simulink model "all_sys_sim"  (R2014a)
settings: Solver=ode45  StartTime=0.0  StopTime=10.0  RelTol=1e-3
values from neighbouring files (symbols this model uses):
  beam_sys = sys_class    [create_all_sys.m]
  build_sys = sys_class    [create_all_sys.m]
  fom_sys = sys_class    [create_all_sys.m]
  heat_sys = sys_class    [create_all_sys.m]
  heli_sys = sys_class    [create_all_sys.m]
  iss_sys = sys_class    [create_all_sys.m]
  mcs_sys = sys_class    [create_all_sys.m]
  MNA1_sys = sys_class    [create_all_sys.m]
  MNA5_sys = sys_class    [create_all_sys.m]
  pde_sys = sys_class    [create_all_sys.m]
  tline_sys = sys_class    [create_all_sys.m]
settings Model: Creator=UX31  LastModifiedBy=UX31

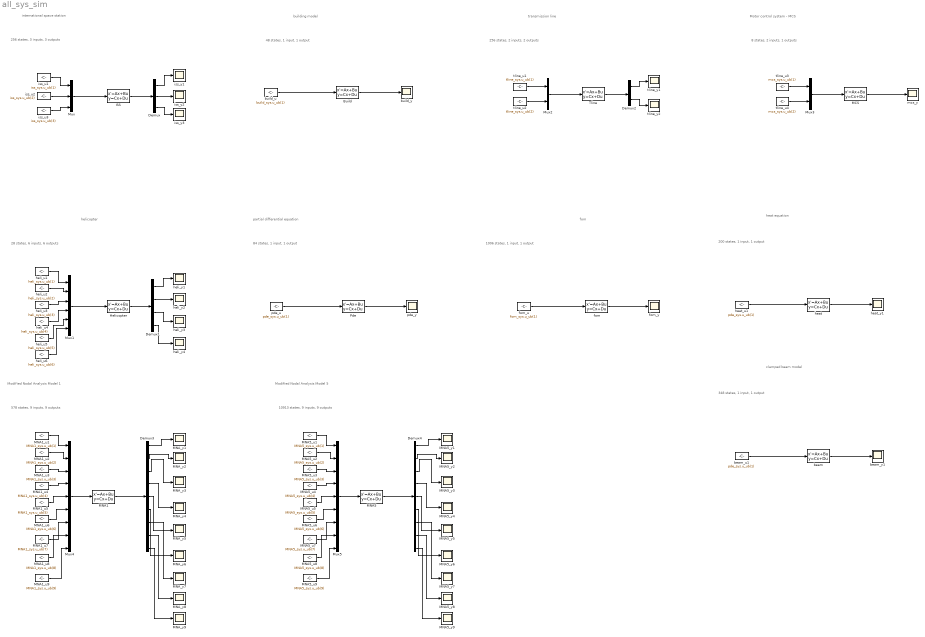
== system all_sys_sim ==
  note: 48 states, 1 input, 1 output
  note: 256 states, 3 inputs, 3 outputs
  note: 84 states, 1 input, 1 output
  note: 28 states, 6 inputs, 6 outputs
  note: 256 states, 2 inputs, 2 outputs
  note: 1006 states, 1 input, 1 output
  note: international space station
  note: building model
  note: helicopter
  note: partial differential equation
  note: fom
  note: transmission line
  note: 8 states, 2 inputs, 1 outputs
  note: Motor control system - MCS
  note: 578 states, 9 inputs, 9 outputs
  note: Modified Nodal Analysis Model 1
  note: 10913 states, 9 inputs, 9 outputs
  note: Modified Nodal Analysis Model 5
  note: 200 states, 1 input, 1 output
  note: heat equation
  note: 348 states, 1 input, 1 output
  note: clamped beam model
  Build : StateSpace  A=build_sys.sys.a  B=build_sys.sys.b  C=build_sys.sys.c  D=build_sys.sys.d  X0=build_sys.x0_lb
  Demux : Demux  Outputs=3
  Demux1 : Demux
  Demux2 : Demux  Outputs=2
  Demux3 : Demux  Outputs=9
  Demux4 : Demux  Outputs=9
  Helicopter : StateSpace  A=heli_sys.sys.a  B=heli_sys.sys.b  C=heli_sys.sys.c  D=heli_sys.sys.d  X0=heli_sys.x0_lb
  ISS : StateSpace  A=iss_sys.sys.a  B=iss_sys.sys.b  C=iss_sys.sys.c  D=iss_sys.sys.d  X0=iss_sys.x0_lb
  MCS : StateSpace  A=mcs_sys.sys.a  B=mcs_sys.sys.b  C=mcs_sys.sys.c  D=mcs_sys.sys.d  X0=mcs_sys.x0_lb
  MNA1 : StateSpace  A=MNA1_sys.sys.a  B=MNA1_sys.sys.b  C=MNA1_sys.sys.c  D=MNA1_sys.sys.d  X0=MNA1_sys.x0_lb
  MNA1_u1 : Constant  Value=MNA1_sys.u_ub(1)
  MNA1_u2 : Constant  Value=MNA1_sys.u_ub(2)
  MNA1_u3 : Constant  Value=MNA1_sys.u_ub(3)
  MNA1_u4 : Constant  Value=MNA1_sys.u_ub(4)
  MNA1_u5 : Constant  Value=MNA1_sys.u_ub(5)
  MNA1_u6 : Constant  Value=MNA1_sys.u_ub(6)
  MNA1_u7 : Constant  Value=MNA1_sys.u_ub(7)
  MNA1_u8 : Constant  Value=MNA1_sys.u_ub(8)
  MNA1_u9 : Constant  Value=MNA1_sys.u_ub(9)
  MNA5 : StateSpace  A=MNA5_sys.sys.a  B=MNA5_sys.sys.b  C=MNA5_sys.sys.c  D=MNA5_sys.sys.d  X0=MNA5_sys.x0_lb
  MNA5_u1 : Constant  Value=MNA5_sys.u_ub(1)
  MNA5_u2 : Constant  Value=MNA5_sys.u_ub(2)
  MNA5_u3 : Constant  Value=MNA5_sys.u_ub(3)
  MNA5_u4 : Constant  Value=MNA5_sys.u_ub(4)
  MNA5_u5 : Constant  Value=MNA5_sys.u_ub(5)
  MNA5_u6 : Constant  Value=MNA5_sys.u_ub(6)
  MNA5_u7 : Constant  Value=MNA5_sys.u_ub(7)
  MNA5_u8 : Constant  Value=MNA5_sys.u_ub(8)
  MNA5_u9 : Constant  Value=MNA5_sys.u_ub(9)
  MNA5_y{1..9} (9 alike) : Scope
      MNA5_y1 settings: SaveName=ScopeData22
      MNA5_y2 settings: SaveName=ScopeData23
      MNA5_y3 settings: SaveName=ScopeData24
      MNA5_y4 settings: SaveName=ScopeData25
      MNA5_y5 settings: SaveName=ScopeData26
      MNA5_y6 settings: SaveName=ScopeData27
      MNA5_y7 settings: SaveName=ScopeData28
      MNA5_y8 settings: SaveName=ScopeData29
      MNA5_y9 settings: SaveName=ScopeData30
  MNA_y{1..9} (9 alike) : Scope
      MNA_y1 settings: SaveName=ScopeData13
      MNA_y2 settings: SaveName=ScopeData14
      MNA_y3 settings: SaveName=ScopeData15
      MNA_y4 settings: SaveName=ScopeData16
      MNA_y5 settings: SaveName=ScopeData17
      MNA_y6 settings: SaveName=ScopeData18
      MNA_y7 settings: SaveName=ScopeData19
      MNA_y8 settings: SaveName=ScopeData20
      MNA_y9 settings: SaveName=ScopeData21
  Mux : Mux  Inputs=3
  Mux1 : Mux  Inputs=6
  Mux2 : Mux  Inputs=2
  Mux3 : Mux  Inputs=2
  Mux4 : Mux  Inputs=9
  Mux5 : Mux  Inputs=9
  Pde : StateSpace  A=pde_sys.sys.a  B=pde_sys.sys.b  C=pde_sys.sys.c  D=pde_sys.sys.d  X0=pde_sys.x0_lb
  Tline : StateSpace  A=tline_sys.sys.a  B=tline_sys.sys.b  C=tline_sys.sys.c  D=tline_sys.sys.d  X0=tline_sys.x0_lb
  beam : StateSpace  A=beam_sys.sys.a  B=beam_sys.sys.b  C=beam_sys.sys.c  D=beam_sys.sys.d  X0=beam_sys.x0_lb
  beam_u1 : Constant  Value=pde_sys.u_ub(1)
  beam_y1 : Scope
      settings: SaveName=ScopeData32
  build_u : Constant  Value=build_sys.u_ub(1)
  build_y : Scope
      settings: SaveName=ScopeData3
  fom : StateSpace  A=fom_sys.sys.a  B=fom_sys.sys.b  C=fom_sys.sys.c  D=fom_sys.sys.d  X0=fom_sys.x0_lb
  fom_u : Constant  Value=fom_sys.u_ub(1)
  fom_y : Scope
      settings: SaveName=ScopeData7
  heat : StateSpace  A=heat_sys.sys.a  B=heat_sys.sys.b  C=heat_sys.sys.c  D=heat_sys.sys.d  X0=heat_sys.x0_lb
  heat_u1 : Constant  Value=pde_sys.u_ub(1)
  heat_y1 : Scope
      settings: SaveName=ScopeData31
  heli_u1 : Constant  Value=heli_sys.u_ub(1)
  heli_u2 : Constant  Value=heli_sys.u_ub(2)
  heli_u3 : Constant  Value=heli_sys.u_ub(3)
  heli_u4 : Constant  Value=heli_sys.u_ub(4)
  heli_u5 : Constant  Value=heli_sys.u_ub(5)
  heli_u6 : Constant  Value=heli_sys.u_ub(6)
  heli_y{1..4} (4 alike) : Scope
      heli_y1 settings: SaveName=ScopeData8
      heli_y2 settings: SaveName=ScopeData9
      heli_y3 settings: SaveName=ScopeData10
      heli_y4 settings: SaveName=ScopeData11
  iss_u1 : Constant  Value=iss_sys.u_ub(1)
  iss_u2 : Constant  Value=iss_sys.u_ub(2)
  iss_u3 : Constant  Value=iss_sys.u_ub(3)
  iss_y1 : Scope
  iss_y2 : Scope
  iss_y3 : Scope
      settings: SaveName=ScopeData2
  mcs_y : Scope
      settings: SaveName=ScopeData12
  pde_u : Constant  Value=pde_sys.u_ub(1)
  pde_y : Scope
      settings: SaveName=ScopeData4
  tline_u1 : Constant  Value=tline_sys.u_ub(1)
  tline_u2 : Constant  Value=tline_sys.u_ub(2)
  tline_u3 : Constant  Value=mcs_sys.u_ub(1)
  tline_u4 : Constant  Value=mcs_sys.u_ub(2)
  tline_y1 : Scope
      settings: SaveName=ScopeData5
  tline_y2 : Scope
      settings: SaveName=ScopeData6
  wires:
  Mux/1 -> ISS/1
  iss_u1/1 -> Mux/1
  iss_u2/1 -> Mux/2
  iss_u3/1 -> Mux/3
  ISS/1 -> Demux/1
  Demux/1 -> iss_y1/1
  Demux/2 -> iss_y2/1
  Demux/3 -> iss_y3/1
  build_u/1 -> Build/1
  Build/1 -> build_y/1
  heli_u1/1 -> Mux1/1
  heli_u2/1 -> Mux1/2
  heli_u3/1 -> Mux1/3
  Mux1/1 -> Helicopter/1
  heli_u4/1 -> Mux1/4
  heli_u5/1 -> Mux1/5
  heli_u6/1 -> Mux1/6
  Helicopter/1 -> Demux1/1
  pde_u/1 -> Pde/1
  Pde/1 -> pde_y/1
  Mux2/1 -> Tline/1
  tline_u1/1 -> Mux2/1
  tline_u2/1 -> Mux2/2
  Tline/1 -> Demux2/1
  Demux2/1 -> tline_y1/1
  Demux2/2 -> tline_y2/1
  fom_u/1 -> fom/1
  fom/1 -> fom_y/1
  Demux1/1 -> heli_y1/1
  Demux1/2 -> heli_y2/1
  Demux1/3 -> heli_y3/1
  Demux1/4 -> heli_y4/1
  Mux3/1 -> MCS/1
  tline_u3/1 -> Mux3/1
  tline_u4/1 -> Mux3/2
  MCS/1 -> mcs_y/1
  MNA1_u1/1 -> Mux4/1
  MNA1_u2/1 -> Mux4/2
  MNA1_u3/1 -> Mux4/3
  Mux4/1 -> MNA1/1
  MNA1_u4/1 -> Mux4/4
  MNA1_u5/1 -> Mux4/5
  MNA1_u6/1 -> Mux4/6
  MNA1/1 -> Demux3/1
  Demux3/1 -> MNA_y1/1
  Demux3/2 -> MNA_y2/1
  Demux3/3 -> MNA_y3/1
  Demux3/4 -> MNA_y4/1
  Demux3/5 -> MNA_y5/1
  Demux3/6 -> MNA_y6/1
  Demux3/7 -> MNA_y7/1
  Demux3/8 -> MNA_y8/1
  Demux3/9 -> MNA_y9/1
  MNA1_u7/1 -> Mux4/7
  MNA1_u8/1 -> Mux4/8
  MNA1_u9/1 -> Mux4/9
  MNA5_u1/1 -> Mux5/1
  MNA5_u2/1 -> Mux5/2
  MNA5_u3/1 -> Mux5/3
  Mux5/1 -> MNA5/1
  MNA5_u4/1 -> Mux5/4
  MNA5_u5/1 -> Mux5/5
  MNA5_u6/1 -> Mux5/6
  MNA5/1 -> Demux4/1
  Demux4/1 -> MNA5_y1/1
  Demux4/2 -> MNA5_y2/1
  Demux4/3 -> MNA5_y3/1
  Demux4/4 -> MNA5_y4/1
  Demux4/5 -> MNA5_y5/1
  Demux4/6 -> MNA5_y6/1
  Demux4/7 -> MNA5_y7/1
  Demux4/8 -> MNA5_y8/1
  Demux4/9 -> MNA5_y9/1
  MNA5_u7/1 -> Mux5/7
  MNA5_u8/1 -> Mux5/8
  MNA5_u9/1 -> Mux5/9
  heat_u1/1 -> heat/1
  heat/1 -> heat_y1/1
  beam_u1/1 -> beam/1
  beam/1 -> beam_y1/1
